simulink library "firstOrderFilter_ul"  (R2020a)
settings: Solver=VariableStepAuto  StartTime=0.0  StopTime=10.0  RelTol=1e-3
settings Model: Creator=mcobb  LastModifiedBy=adabney
settings DataIOCC: ReturnWorkspaceOutputs=off
settings DebuggingCC: ArithmeticOperatorsInVariantConditions=warning
settings SFSimCC: CustomCodeUndefinedFunction=UseInterfaceOnly

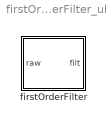
== system firstOrderFilter_ul ==
  firstOrderFilter : Subsystem  TreatAsAtomicUnit=on  mask{tau=0, ic=0}
      mask prompts: tau "Time Const [s]"; ic "Initial Condition"
      settings: MinAlgLoopOccurrences=on

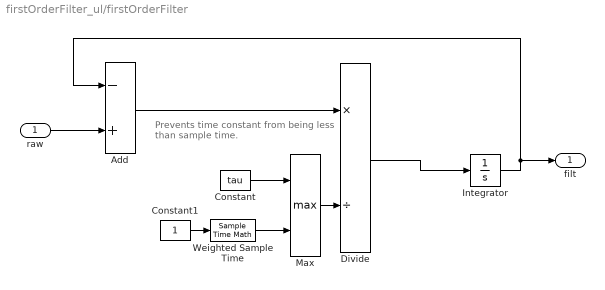
== system firstOrderFilter_ul/firstOrderFilter ==
  note: Prevents time constant from
      | being less than sample time.
  raw : Inport
  Add : Sum  Inputs=-+
  Constant : Constant  Value=tau
  Constant1 : Constant
  Divide : Product  Inputs=*/
  Integrator : Integrator  InitialCondition=ic
  Max : MinMax  Function=max  Inputs=2
  Weighted Sample Time : SampleTimeMath  TsampMathOp=Ts Only
  filt : Outport  VectorParamsAs1DForOutWhenUnconnected=off
  wires:
  raw/1 -> Add/2
  Add/1 -> Divide/1
  Max/1 -> Divide/2
  Constant/1 -> Max/1
  Constant1/1 -> Weighted Sample Time/1
  Weighted Sample Time/1 -> Max/2
  Divide/1 -> Integrator/1
  Integrator/1 -> Add/1, filt/1
